simulink model "chap8_11sim"  (R2015a)
settings: Solver=ode45  StartTime=0.0  StopTime=100  RelTol=1e-3
settings Model: Creator=zhr  LastModifiedBy=zhr

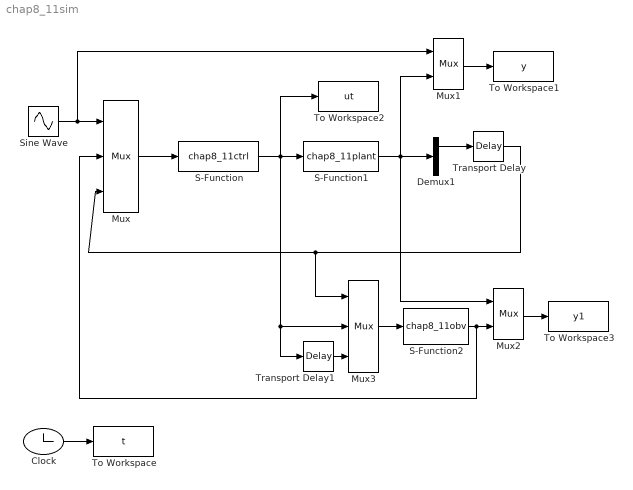
== system chap8_11sim ==
  Clock : Clock
  Demux1 : Demux  Outputs=2
  Mux : Mux  Inputs=3
  Mux1 : Mux  Inputs=2
  Mux2 : Mux  Inputs=2
  Mux3 : Mux  Inputs=3
  S-Function : S-Function  FunctionName=chap8_11ctrl
  S-Function1 : S-Function  FunctionName=chap8_11plant
  S-Function2 : S-Function  FunctionName=chap8_11obv
  Sine Wave : Sin  SampleTime=0
  To Workspace : ToWorkspace  VariableName=t  SampleTime=-1
  To Workspace1 : ToWorkspace  VariableName=y  SampleTime=-1
  To Workspace2 : ToWorkspace  VariableName=ut  SampleTime=-1
  To Workspace3 : ToWorkspace  VariableName=y1  SampleTime=-1
  Transport Delay : TransportDelay
  Transport Delay1 : TransportDelay
  wires:
  Clock/1 -> To Workspace/1
  Sine Wave/1 -> Mux1/1, Mux/1
  Mux/1 -> S-Function/1
  S-Function/1 -> Mux3/2, Transport Delay1/1, To Workspace2/1, S-Function1/1
  S-Function1/1 -> Mux1/2, Mux2/1, Demux1/1
  Demux1/1 -> Transport Delay/1
  Transport Delay/1 -> Mux3/1, Mux/3
  Mux1/1 -> To Workspace1/1
  Transport Delay1/1 -> Mux3/3
  Mux3/1 -> S-Function2/1
  S-Function2/1 -> Mux/2, Mux2/2
  Mux2/1 -> To Workspace3/1
